simulink subsystem "starSensorMeasure"  (R2024b)
settings: Solver=VariableStepAuto  StartTime=0.0  StopTime=10.0  RelTol=1e-3
undefined symbols (not defined in the file): sensors
libraries: matrix_library x1
settings Model: Creator=ricca  LastModifiedBy=ricca

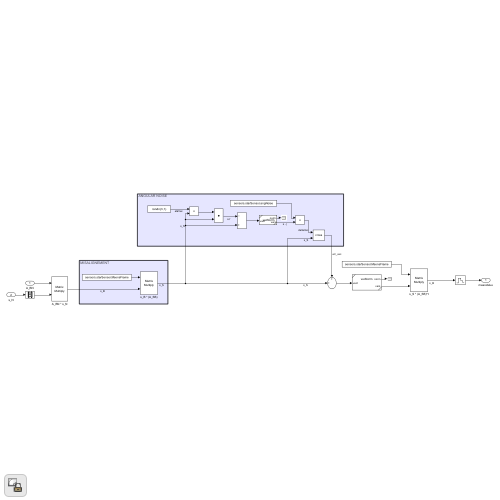
[thumbnail: Simulink's stored preview of the top-level diagram]
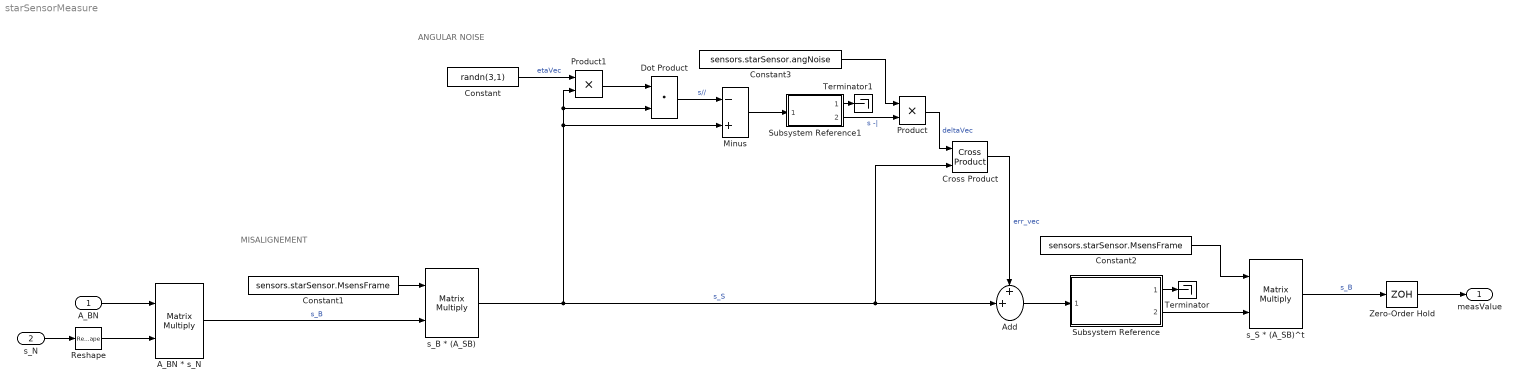
== system starSensorMeasure ==
  note: ANGULAR NOISE
  note: MISALIGNEMENT
  A_BN : Inport
  s_N : Inport  Port=2
  A_BN * s_N : Product  Multiplication=Matrix(*)
  Add : Sum  Inputs=++|
  Constant : Constant  Value=randn(3,1)
  Constant1 : Constant  Value=sensors.starSensor.MsensFrame
  Constant2 : Constant  Value=sensors.starSensor.MsensFrame
  Constant3 : Constant  Value=sensors.starSensor.angNoise
  Cross Product : matrix_library/Cross Product
  Dot Product : DotProduct  OutDataTypeStr=Inherit: Inherit via internal rule
  Minus : Sum  Inputs=-+
  Product : Product
  Product1 : Product
  Reshape : Reshape  OutputDimensionality=Column vector (2-D)
  Subsystem Reference : Subsystem  ReferencedSubsystem=vecNorm
  Subsystem Reference1 : Subsystem  ReferencedSubsystem=vecNorm
  Terminator : Terminator
  Terminator1 : Terminator
  Zero-Order Hold : ZeroOrderHold  SampleTime=sensors.starSensor.sampleTime
  s_B * (A_SB) : Product  Multiplication=Matrix(*)
  s_S * (A_SB)^t : Product  Multiplication=Matrix(*)
  measValue : Outport
  wires:
  s_B * (A_SB)/1 -> Add/2, Cross Product/2, Product1/2, Dot Product/2, Minus/2  "s_S"
  Subsystem Reference/2 -> s_S * (A_SB)^t/2
  Subsystem Reference/1 -> Terminator/1
  Constant1/1 -> s_B * (A_SB)/1
  A_BN * s_N/1 -> s_B * (A_SB)/2  "s_B"
  A_BN/1 -> A_BN * s_N/1
  Constant/1 -> Product1/1  "etaVec"
  Cross Product/1 -> Add/1  "err_vec"
  Constant2/1 -> s_S * (A_SB)^t/1
  s_S * (A_SB)^t/1 -> Zero-Order Hold/1  "s_B"
  Add/1 -> Subsystem Reference/1
  Product1/1 -> Dot Product/1
  Dot Product/1 -> Minus/1  "s//"
  Subsystem Reference1/1 -> Terminator1/1
  Minus/1 -> Subsystem Reference1/1
  Subsystem Reference1/2 -> Product/2  "s -|"
  Constant3/1 -> Product/1
  Product/1 -> Cross Product/1  "deltaVec"
  s_N/1 -> Reshape/1
  Zero-Order Hold/1 -> measValue/1
  Reshape/1 -> A_BN * s_N/2
